simulink model "sumpModelWaterOnly"  (R2019a)
settings: Solver=VariableStepAuto  StartTime=0.0  StopTime=10.0  RelTol=1e-3
settings Model: Creator=jason.miskin  LastModifiedBy=jason.miskin
settings DataIOCC: ExternalInput=[t, u1,u2,u3]  LoadExternalInput=on

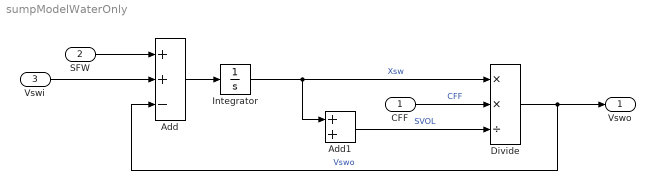
== system sumpModelWaterOnly ==
  CFF : Inport
  SFW : Inport  Port=2
  Vswi : Inport  Port=3
  Add : Sum  Inputs=++-
  Add1 : Sum
  Divide : Product  Inputs=**/
  Integrator : Integrator  InitialCondition=15
  Vswo : Outport
  wires:
  CFF/1 -> Divide/2  "CFF"
  Add1/1 -> Divide/3  "SVOL"
  Integrator/1 -> Add1/1, Divide/1  "Xsw"
  ? -> Add1/2  "Xss"
  SFW/1 -> Add/1
  Vswi/1 -> Add/2
  Add/1 -> Integrator/1
  Divide/1 -> Add/3, Vswo/1  "Vswo"
